simulink model "Block_SetHandout"  (R2021a)
settings: Solver=FixedStepAuto  StartTime=0.0  StopTime=inf  FixedStep=1/100  RelTol=1e-3
settings Model: EnablePacing=on  PacingRate=13  Creator=Peska  LastModifiedBy=Peska

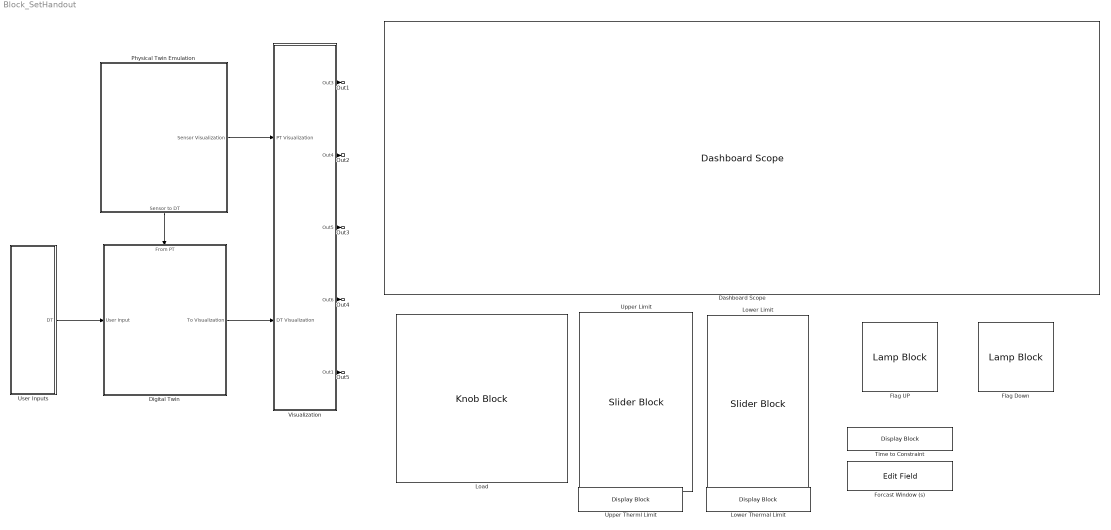
== system Block_SetHandout ==
  " Time to Constraint" : DisplayBlock  LabelPosition=Hide  Format=short  Transparency=1
  Dashboard Scope : DashboardScope  TimeSpan=50  Ymin=22  Ymax=27  UpdateMode=Scroll
  Digital Twin : Subsystem
      settings: PortSchema="{\"entries\":[{\"content\":{\"sides\":[{\"content\":{\"connectorIds\":[\"Out1\"]},\"type\":\"ConnectorPlacement.EquallySpacedRectSide\",\"uuid\":\"677e82ea-ff82-4c96-90ba-310ae7642166\"},{\"content\":{\"connectorIds\":[\"In2\"],\"side\":\"RIGHT\"},\"type\":\"ConnectorPlacement.EquallySpacedRectSide\",\"uuid\":\"566a3afd-bfe2-470e-b0e0-0e84e53a5785\"},{\"content\":{\"connectorIds\":[\"In1\"],\"side\":\"TOP\"},\"type\":\"ConnectorPlacement.EquallySpacedRectSide\",\"uuid\":\"2c377fd5-b6e8-4a8d-918f-b3caf8f79c5a\"}]},\"type\":\"ConnectorPlacement.EquallySpacedConnector\",\"uuid\":\"392c3050-1701-4dfe-a9ac-94477734c3cd\"}],\"packageUris\":[\"http://schema.mathworks.com/mf0/Connector/R2020b\"],\"version\":\"1.0\"}"
  Flag Down : LampBlock  LabelPosition=Hide
  Flag UP : LampBlock  LabelPosition=Hide
  Forcast Window (s) : EditField  LabelPosition=Hide  ShowInitialText=on  Alignment=Center
  Load : KnobBlock  LabelPosition=Hide  ScaleMax=7  TickInterval=1
  Lower Limit : SliderBlock  LabelPosition=Hide  ScaleMin=20  ScaleMax=80  TickInterval=10
  Lower Thermal Limit : DisplayBlock  LabelPosition=Hide  Format=shortG  Transparency=1
  Physical Twin Emulation : Subsystem
      settings: PortSchema="{\"entries\":[{\"content\":{\"sides\":[{\"content\":{\"connectorIds\":[]},\"type\":\"ConnectorPlacement.EquallySpacedRectSide\",\"uuid\":\"677e82ea-ff82-4c96-90ba-310ae7642166\"},{\"content\":{\"connectorIds\":[\"Out1\"],\"side\":\"RIGHT\"},\"type\":\"ConnectorPlacement.EquallySpacedRectSide\",\"uuid\":\"566a3afd-bfe2-470e-b0e0-0e84e53a5785\"},{\"content\":{\"connectorIds\":[],\"side\":\"TOP\"},\"type\":\"ConnectorPlacement.EquallySpacedRectSide\",\"uuid\":\"2c377fd5-b6e8-4a8d-918f-b3caf8f79c5a\"},{\"content\":{\"connectorIds\":[\"Out2\"],\"side\":\"BOTTOM\"},\"type\":\"ConnectorPlacement.EquallySpacedRectSide\",\"uuid\":\"18b914a8-5a07-4a5d-9870-c18a293ad2d0\"}]},\"type\":\"ConnectorPlacement.EquallySpacedConnector\",\"uuid\":\"392c3050-1701-4dfe-a9ac-94477734c3cd\"}],\"packageUris\":[\"http://schema.mathworks.com/mf0/Connector/R2020b\"],\"version\":\"1.0\"}"
  Upper Limit : SliderBlock  LabelPosition=Hide  ScaleMin=20  ScaleMax=80  TickInterval=10
  Upper Therml Limit : DisplayBlock  LabelPosition=Hide  Format=shortG  Transparency=1
  User Inputs : Subsystem
  Visualization : Subsystem
  Out1 : Outport
  Out2 : Outport  Port=2
  Out3 : Outport  Port=3
  Out4 : Outport  Port=4
  Out5 : Outport  Port=5
  wires:
  Digital Twin/1(To Visualization) -> Visualization/2(DT Visualization)
  User Inputs/1(DT) -> Digital Twin/2(User Input)
  Physical Twin Emulation/1("Sensor Visualization ") -> Visualization/1("PT Visualization ")
  Physical Twin Emulation/2(Sensor to DT) -> Digital Twin/1(From PT)
  Visualization/1(Out3) -> Out1/1
  Visualization/2(Out4) -> Out2/1
  Visualization/3(Out5) -> Out3/1
  Visualization/4(Out6) -> Out4/1
  Visualization/5(Out1) -> Out5/1

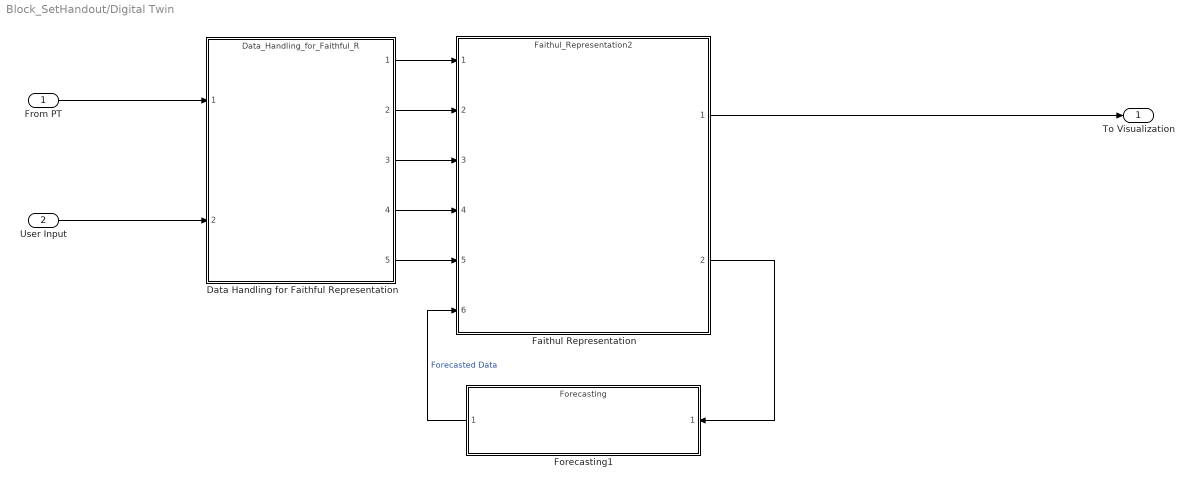
== system Block_SetHandout/Digital Twin ==
  From PT : Inport
  User Input : Inport  Port=2
  Data Handling for Faithful Representation : ModelReference  ModelNameDialog=Data_Handling_for_Faithful_R.slxp  ModelReferenceVersion=1.6  CopyOfModelProtected=on
  Faithul Representation : ModelReference  ModelNameDialog=Faithul_Representation2.slxp  ModelReferenceVersion=1.10  CopyOfModelProtected=on
  Forecasting1 : ModelReference  ModelNameDialog=Forecasting.slxp  ModelReferenceVersion=1.4  CopyOfModelProtected=on
  To Visualization : Outport
  wires:
  User Input/1 -> Data Handling for Faithful Representation/2
  Forecasting1/1 -> Faithul Representation/6  "Forecasted Data"
  From PT/1 -> Data Handling for Faithful Representation/1
  Data Handling for Faithful Representation/1 -> Faithul Representation/1
  Data Handling for Faithful Representation/3 -> Faithul Representation/3
  Data Handling for Faithful Representation/5 -> Faithul Representation/5
  Data Handling for Faithful Representation/4 -> Faithul Representation/4
  Data Handling for Faithful Representation/2 -> Faithul Representation/2
  Faithul Representation/1 -> To Visualization/1
  Faithul Representation/2 -> Forecasting1/1

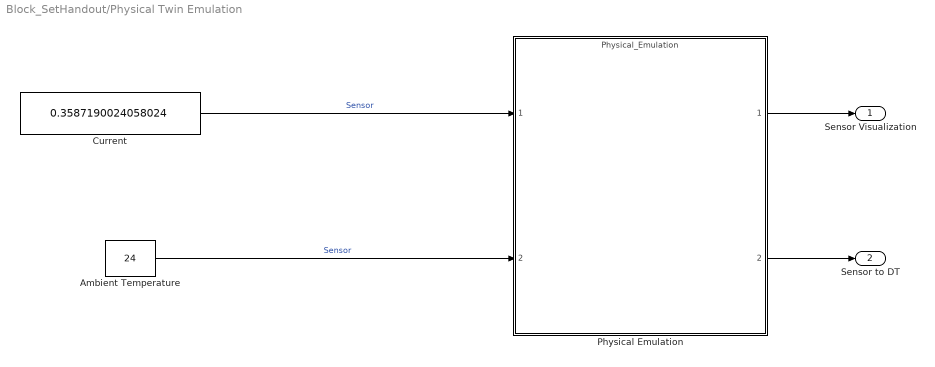
== system Block_SetHandout/Physical Twin Emulation ==
  Ambient Temperature : Constant  Value=24
  Current : Constant  Value=0.3587190024058024
  Physical Emulation : ModelReference  ModelNameDialog=Physical_Emulation.slxp  ModelReferenceVersion=1.6  CopyOfModelProtected=on
  "Sensor Visualization " : Outport
  Sensor to DT : Outport  Port=2
  wires:
  Physical Emulation/1 -> "Sensor Visualization "/1
  Physical Emulation/2 -> Sensor to DT/1
  Current/1 -> Physical Emulation/1  "Sensor"
  Ambient Temperature/1 -> Physical Emulation/2  "Sensor"

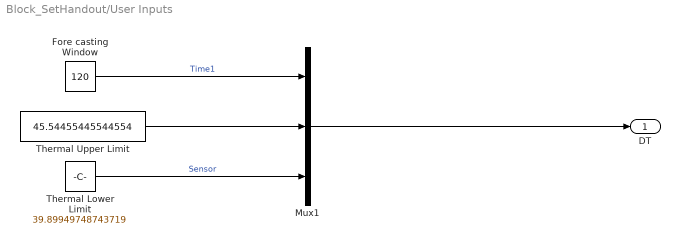
== system Block_SetHandout/User Inputs ==
  Fore casting Window : Constant  Value=120
  Mux1 : Mux  Inputs=3
  Thermal Lower Limit : Constant  Value=39.89949748743719
  Thermal Upper Limit : Constant  Value=45.54455445544554
  DT : Outport
  wires:
  Fore casting Window/1 -> Mux1/1  "Time1"
  Thermal Upper Limit/1 -> Mux1/2
  Thermal Lower Limit/1 -> Mux1/3  "Sensor"
  Mux1/1 -> DT/1

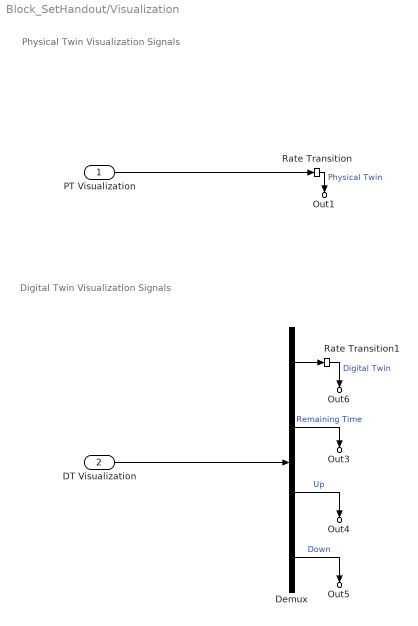
== system Block_SetHandout/Visualization ==
  note: Digital Twin Visualization Signals
  note: Physical Twin Visualization Signals
  "PT Visualization " : Inport
  DT Visualization : Inport  Port=2
  Demux : Demux
  Rate Transition : RateTransition  OutPortSampleTime=1
  Rate Transition1 : RateTransition  OutPortSampleTime=1
  Out3 : Outport
  Out4 : Outport  Port=2
  Out5 : Outport  Port=3
  Out6 : Outport  Port=4
  Out1 : Outport  Port=5
  wires:
  Demux/3 -> Out4/1  "Up"
  Rate Transition1/1 -> Out6/1  "Digital Twin"
  Demux/2 -> Out3/1  "Remaining Time"
  Demux/4 -> Out5/1  "Down"
  DT Visualization/1 -> Demux/1
  Demux/1 -> Rate Transition1/1
  Rate Transition/1 -> Out1/1  "Physical Twin"
  "PT Visualization "/1 -> Rate Transition/1
